simulink model "ArmTest2"  (R2023a)
settings: Solver=VariableStepAuto  StartTime=0.0  StopTime=50  RelTol=1e-3
libraries: dspnetwork x2
settings Model: Creator=skala  LastModifiedBy=jeric
settings ModelReferenceCC: EnableRefExpFcnMdlSchedulingChecks=on

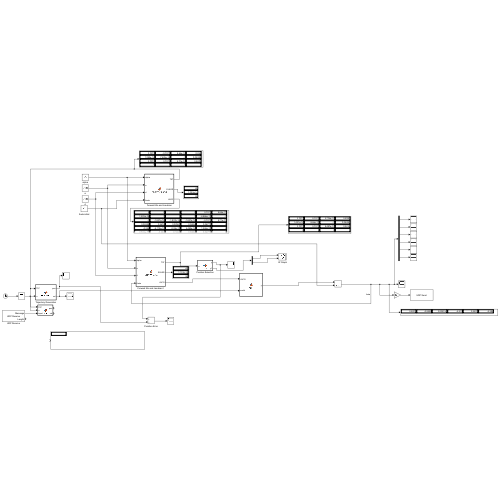
[thumbnail: Simulink's stored preview of the top-level diagram]
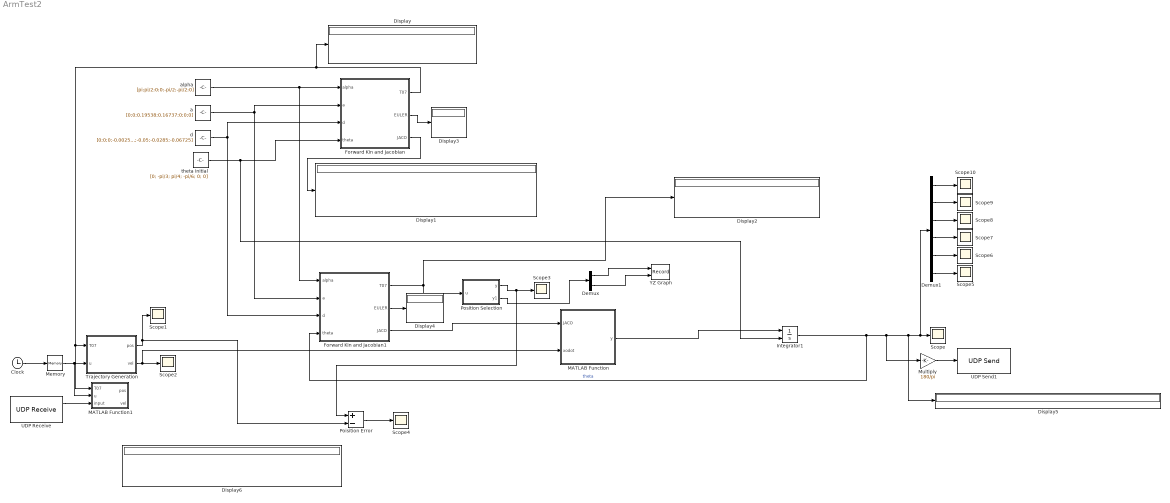
== system ArmTest2 ==
  Clock : Clock
  Demux : Demux  Outputs=2
  Demux1 : Demux  Outputs=6
  Display{,1..6} (7 alike) : Display
  Forward Kin and Jacobian : MATLAB Function  TreatAsAtomicUnit=on
  Forward Kin and Jacobian1 : MATLAB Function  TreatAsAtomicUnit=on
  Integrator1 : Integrator  InitialConditionSource=external  InitialCondition=[pi/2;0;-pi/2;pi/6;0;pi/4]
  MATLAB Function : MATLAB Function  TreatAsAtomicUnit=on
  MATLAB Function1 : MATLAB Function  TreatAsAtomicUnit=on
  Memory : Memory  InheritSampleTime=on
  Multiply : Gain  Gain=180/pi
  Poisition Error : Sum  Inputs=+-
  Position Selection : MATLAB Function  TreatAsAtomicUnit=on
  Scope{,1..10} (11 alike) : Scope
  Trajectory Generation : MATLAB Function  TreatAsAtomicUnit=on
  UDP Receive : dspnetwork/UDP Receive  localURL='0.0.0.0'  localPort=28008  remoteURL='127.0.0.1'  remotePort=-1  recvBufferSize=2500  dims=24  signalDatatype=double  isComplex=off  isVarSize=off  showBlockingTime=off  blockingTime=0  sampletime=.0001  blockPlatform=[]
      settings: LibrarySourceBlock=dspsrcs4/UDP Receive
  UDP Send1 : dspnetwork/UDP Send  remoteURL='127.0.0.1'  remotePort=28007  localURL='0.0.0.0'  localPortSource=Automatically determine  localPort=-1  sendBufferSize=8192  sampletime=-1  blockPlatform=[]  separateLengthPort=0
      settings: LibrarySourceBlock=dspsnks4/UDP Send
  YZ Graph : Record  FileSettingsInternal="{\"entries\":[{\"content\":{\"excelSettings\":{\"content\":{},\"type\":\"Streamout.ExcelSettings\"}},\"type\":\"Streamout.FileSettingStorage\",\"uuid\":\"\"}],\"packageUris\":[\"http:\\/\\/schema.mathworks.com\\/mf0\\/streamout_blocks\\/R2020a\"],\"version\":\"1.0\"}"  Layout=[1 1]  SignalsInternal="{\"entries\":[{\"content\":{\"signals\":[{\"content\":{\"blockPath\":[],\"dimensions\":[1,1],\"domain\":\"\",\"lineColor\":\"#0072bd\",\"plots\":[1],\"port\":1,\"sid\":[\"\"],\"signalID\":3755,\"signalName\":\"Demux:1\"},\"type\":\"RecordBlkView.Signal\",\"uuid\":\"\"},{\"content\":{\"blockPath\":[],\"dimensions\":[1,1],\"domain\":\"\",\"lineColor\":\"#d95319\",\"plots\":[1],\"port\":2,\"sid\":[\"\"],\"signalID\":3759,\"signalName\":\"Demux:2\"},\"type\":\"RecordBlkView.Signal\",\"uuid\":\"\"}]},\"type\":\"RecordBlkView.InputSignals\",\"uuid\":\"\"}],\"packageUris\":[\"http:\\/\\/schema.mathworks.com\\/mf0\\/streamout_blocks\\/R2020a\"],\"version\":\"1.0\"}"  VisualizationBindings="{\"xyplotplugin\":{\"info\":[{\"series\":[{\"bindingParametersList\":[{\"parameter\":\"Y-Axis\",\"signalID\":3759,\"signalName\":\"Demux:2\"},{\"parameter\":\"X-Axis\",\"signalID\":3755,\"signalName\":\"Demux:1\"}],\"seriesID\":32003}],\"subplotID\":1}]}}"  CompatibilityTag=XY
  a : Constant  Value=[0;0;0.19538;0.16737;0;0;0]
  alpha : Constant  Value=[pi;pi/2;0;0;-pi/2;-pi/2;0]
  d : Constant  Value=[0;0;0;-0.0025;-0.05;-0.0285;-0.06725]
  theta initial : Constant  Value=[0; -pi/3; pi/4; -pi/6; 0; 0]
  wires:
  alpha/1 -> Forward Kin and Jacobian1/1(alpha), Forward Kin and Jacobian/1(alpha)
  a/1 -> Forward Kin and Jacobian1/2(a), Forward Kin and Jacobian/2(a)
  d/1 -> Forward Kin and Jacobian1/3(d), Forward Kin and Jacobian/3(d)
  Integrator1/1 -> Forward Kin and Jacobian1/4(theta), Multiply/1, Display5/1, Demux1/1, Scope/1  "theta"
  theta initial/1 -> Integrator1/2, Forward Kin and Jacobian/4(theta)
  Forward Kin and Jacobian/1(T07) -> MATLAB Function1/1(T07), Trajectory Generation/1(T07), Display/1
  Forward Kin and Jacobian/3(JACO) -> Display1/1
  Trajectory Generation/2(vel) -> MATLAB Function/2(xodot), Scope2/1
  Clock/1 -> Memory/1
  Forward Kin and Jacobian1/3(JACO) -> MATLAB Function/1(JACO)
  MATLAB Function/1(y) -> Integrator1/1
  Forward Kin and Jacobian1/1(T07) -> Position Selection/1(u), Display2/1
  Position Selection/1(y) -> Poisition Error/1, Scope3/1
  Trajectory Generation/1(pos) -> Poisition Error/2, Scope1/1
  Poisition Error/1 -> Scope4/1
  Forward Kin and Jacobian/2(EULER) -> Display3/1
  Forward Kin and Jacobian1/2(EULER) -> Display4/1
  Demux/2 -> YZ Graph/2
  Position Selection/2(y1) -> Demux/1
  Demux/1 -> YZ Graph/1
  Multiply/1 -> UDP Send1/1
  Memory/1 -> MATLAB Function1/2(u), Trajectory Generation/2(u)
  Demux1/6 -> Scope5/1
  Demux1/5 -> Scope6/1
  Demux1/4 -> Scope7/1
  Demux1/1 -> Scope10/1
  Demux1/2 -> Scope9/1
  Demux1/3 -> Scope8/1
  UDP Receive/1 -> MATLAB Function1/3(input)

== matlab function ArmTest2/Forward Kin and Jacobian1 ==
  data: alpha input; T07 output; EULER output; a input; d input; theta input; JACO output
function [T07,EULER,JACO]= FORWANDJAC(alpha,a,d,theta)
%theta1=theta(1); theta2=theta(2); theta3=theta(3); 
%theta4=theta(4); theta5= theta(5); theta6=theta(6); 

P=[0;0;1];
%
T01=DHPM(alpha(1),a(1),d(1),theta(1));
e1=T01(1:3,1:3)*P;
%
T12=DHPM(alpha(2),a(2),d(2), theta(2));
T02=T01*T12;
e2=T02(1:3,1:3)*P;
%
T23=DHPM(alpha(3), a(3),d(3), theta(3));
T03=T02*T23;
e3=T03(1:3,1:3)*P;
%
T34=DHPM(alpha(4), a(4),d(4), theta(4));
T04=T03*T34;
e4=T04(1:3,1:3)*P;
%
T45=DHPM(alpha(5), a(5),d(5), theta(5));
T05=T04*T45;
e5=T05(1:3,1:3)*P;
%
T56=DHPM(alpha(6),a(6),d(6), theta(6)) ;
T06=T05*T56;
e6=T06(1:3,1:3)*P;
%
T67=DHPM(alpha(7), a(7),d(7),0);
T07=T06*T67;
P67L=T67(1:3,4);
P67=T07(1:3,1:3)*P67L;
%
T57=T56*T67;
P57L=T57(1:3,4);
P57=T05(1:3,1:3)*P57L;
%
T47=T45*T57;
P47L=T47(1:3,4);
P47=T04(1:3,1:3)*P47L;
%
T37=T34*T47;
P37L=T37(1:3,4);
P37=T03(1:3,1:3)*P37L;
%
T27=T23*T37;
P27L=T27(1:3,4);
P27=T02(1:3,1:3)*P27L;
%
T17=T12*T27;
P17L=T17(1:3,4);
P17=T01(1:3,1:3)*P17L;
%
T07=T01*T17;
P07=T07(1:3,4);
%
  beta=atan2(-T07(3,1),sqrt(T07(1,1)^2+T07(2,1)^2));
  if beta == pi/2
     alph=0.0;
     gamma=atan2(T07(1,2),T07(2,2));
  elseif beta==-pi/2
      alph=0.0;
      gamma=-atan2(T07(1,2),T07(2,2));
  else
  cb=cos(beta);
  alph=atan2(T07(2,1)/cb, T07(1,1)/cb);
  gamma=atan2(T07(3,2)/cb, T07(3,3)/cb);
  end
  EULER=[beta;alph;gamma]*180/pi;
%
JACT=[e1,e2,e3,e4,e5,e6];
b1=cross(e1,P17);
b2=cross(e2,P27);
b3=cross(e3,P37);
b4=cross(e4,P47);
b5=cross(e5,P57);
b6=cross(e6,P67);
JACB=[b1,b2,b3,b4,b5,b6];
JACO=[JACT;JACB];



function T=DHPM(alpha, a, d, theta)

T_xAlpha=[1 0 0 0 ;0 cos(alpha) -sin(alpha) 0 ;0 sin(alpha) cos(alpha) 0;0 0 0 1];
T_xA=[1 0 0 a;0 1 0 0;0 0 1 0;0 0 0 1];
T_zD=[1 0 0 0;0 1 0 0;0 0 1 d;0 0 0 1];
T_zTheta=[cos(theta) -sin(theta) 0 0;sin(theta) cos(theta) 0 0;0 0 1 0;0 0 0 1];
T=T_xAlpha*T_xA*T_zD*T_zTheta;

== matlab function ArmTest2/Trajectory Generation ==
  data: T07 input; u input; pos output; vel output
function [pos,vel] = TRAJGEN(T07, u)

omega=2*pi/5;
r=sqrt(T07(2,4)^2+T07(3,4)^2);
beta1=atan2(T07(3,4),T07(2,4));
xx=T07(1,4);
zz=r*sin(omega*u+beta1);
yy=r*cos(omega*u+beta1);
xxdot=0;
yydot=-r*omega*sin(omega*u+beta1);
zzdot=r*omega*cos(omega*u+beta1);
xodot=[zeros(4,1);yydot;zzdot];
%xo=T07;
%x1=T07(1:3,4);
vel =xodot;
pos=[xx;yy;zz];

== matlab function ArmTest2/Forward Kin and Jacobian ==
  data: alpha input; T07 output; EULER output; a input; d input; theta input; JACO output
function [T07,EULER,JACO]= FORWANDJAC(alpha,a,d,theta)
%theta1=theta(1); theta2=theta(2); theta3=theta(3); 
%theta4=theta(4); theta5= theta(5); theta6=theta(6); 
P=[0;0;1];
%
T01=DHPM(alpha(1),a(1),d(1),theta(1));
e1=T01(1:3,1:3)*P;
%
T12=DHPM(alpha(2),a(2),d(2), theta(2));
T02=T01*T12;
e2=T02(1:3,1:3)*P;
%
T23=DHPM(alpha(3), a(3),d(3), theta(3));
T03=T02*T23;
e3=T03(1:3,1:3)*P;
%
T34=DHPM(alpha(4), a(4),d(4), theta(4));
T04=T03*T34;
e4=T04(1:3,1:3)*P;
%
T45=DHPM(alpha(5), a(5),d(5), theta(5));
T05=T04*T45;
e5=T05(1:3,1:3)*P;
%
T56=DHPM(alpha(6),a(6),d(6), theta(6)) ;
T06=T05*T56;
e6=T06(1:3,1:3)*P;
%
T67=DHPM(alpha(7), a(7),d(7),0);
T07=T06*T67;
P67L=T67(1:3,4);
P67=T07(1:3,1:3)*P67L;
%
T57=T56*T67;
P57L=T57(1:3,4);
P57=T05(1:3,1:3)*P57L;
%
T47=T45*T57;
P47L=T47(1:3,4);
P47=T04(1:3,1:3)*P47L;
%
T37=T34*T47;
P37L=T37(1:3,4);
P37=T03(1:3,1:3)*P37L;
%
T27=T23*T37;
P27L=T27(1:3,4);
P27=T02(1:3,1:3)*P27L;
%
T17=T12*T27;
P17L=T17(1:3,4);
P17=T01(1:3,1:3)*P17L;
%
T07=T01*T17;
P07=T07(1:3,4);
  beta=atan2(-T07(3,1),sqrt(T07(1,1)^2+T07(2,1)^2));
  if beta==pi/2
     alph=0.0;
     gamma=atan2(T07(1,2),T07(2,2));
  elseif beta==-pi/2
      alph=0.0;
      gamma=-atan2(T07(1,2),T07(2,2));
  else
  cb=cos(beta);
  alph=atan2(T07(2,1)/cb, T07(1,1)/cb);
  gamma=atan2(T07(3,2)/cb, T07(3,3)/cb);
  end
  EULER=[beta;alph;gamma]*180/pi;

JACT=[e1,e2,e3,e4,e5,e6];
b1=cross(e1,P17);
b2=cross(e2,P27);
b3=cross(e3,P37);
b4=cross(e4,P47);
b5=cross(e5,P57);
b6=cross(e6,P67);
JACB=[b1,b2,b3,b4,b5,b6];
JACO=[JACT;JACB];



function T=DHPM(alpha, a, d, theta)

T_xAlpha=[1 0 0 0 ;0 cos(alpha) -sin(alpha) 0 ;0 sin(alpha) cos(alpha) 0;0 0 0 1];
T_xA=[1 0 0 a;0 1 0 0;0 0 1 0;0 0 0 1];
T_zD=[1 0 0 0;0 1 0 0;0 0 1 d;0 0 0 1];
T_zTheta=[cos(theta) -sin(theta) 0 0;sin(theta) cos(theta) 0 0;0 0 1 0;0 0 0 1];
T=T_xAlpha*T_xA*T_zD*T_zTheta;

== matlab function ArmTest2/MATLAB Function ==
  data: JACO input; xodot input; y output
function y = fcn(JACO, xodot)
%thetadot=JACO\xodot;
thetadot=JACO\xodot;
y=thetadot;

== matlab function ArmTest2/Position Selection ==
  data: u input; y output; y1 output
function [y, y1] = fcn(u)
pos1=u(1:3,4);
y = pos1;
y1=u(2:3,4);

== matlab function ArmTest2/MATLAB Function1 ==
  data: T07 input; u input; pos output; vel output; input input
function [pos, vel] = fcn(T07, u, input)

dir = input(19 : 21);

xini = T07(1 : 3, 4);
v = 0.01;
magdir = sqrt(dir(1) ^ 2 + dir(2) ^ 2 + dir(3) ^ 2);
val = v * dir / magdir;

xdot = [zeros(3, 1); val];

pos = xini + val * u;
vel = xdot;
